simulink model "Tractive_System_model"  (R2025b)
settings: Solver=ode15s  StartTime=0  StopTime=85  MaxStep=1e-5  MinStep=1e-8  RelTol=1e-3  AbsTol=1e-6
undefined symbols (not defined in the file): FL, FR, RL, RR
libraries: batteryecm_lib x280, fl_lib x60, nesl_utility x36, ee_lib x9, sdl_lib x9, simulink x1, slpidlib x1, autolibshared x1, eePmsmFieldOrientedControl x1, eePmsmFwController x1
(part 23 of 23)

== system Tractive_System_model/Electric Powertrain/Scopes Motor/losses ==
  idq : Inport
  w : Inport  Port=2
  Constant : Constant  Value=666.7
  Constant1 : Constant  Value=0.0393
  Constant2 : Constant  Value=[0.695, 8.35e-4, 5.37e-3]  OutDataTypeStr=double
  Constant3 : Constant  Value=[0.298, 3.58e-4, 2.30e-3]  OutDataTypeStr=double
  MATLAB Function : MATLAB Function  TreatAsAtomicUnit=on
  tq_loss : Outport
  wires:
  w/1 -> MATLAB Function/2(w)
  MATLAB Function/1(trq_loss) -> tq_loss/1
  idq/1 -> MATLAB Function/1(idq)
  Constant/1 -> MATLAB Function/4(f_losses)
  Constant1/1 -> MATLAB Function/3(PM)
  Constant2/1 -> MATLAB Function/5(losses_oc)
  Constant3/1 -> MATLAB Function/6(losses_sc)

== system Tractive_System_model/Electric Powertrain/Thermal model/Sensing Temperature Rot ==
  PS-Simulink Converter : nesl_utility/PS-Simulink Converter  PhysicalDomain=network_engine_domain  SubClassName=ps_output  LeftPortType=input  RightPortType=output  PseudoPeriodic=off  Frequencies=[]  VectorFormat=1-D array  Unit=degC  AffineConversion=on
  Temperature Sensor : fl_lib/Thermal/Thermal Sensors/Temperature Sensor  temperature_measure=foundation.enum.MeasurementReference.difference
  ThRef : fl_lib/Thermal/Thermal Elements/Thermal Reference
  H : PMIOPort  Side=Left
  tag scope: TR=global
  wires:
  PS-Simulink Converter/1 -> [TR]
  connections:
  Temperature Sensor/RConn2 -- PS-Simulink Converter/LConn1
  ThRef/LConn1 -- Temperature Sensor/RConn1
  H/RConn1 -- Temperature Sensor/LConn1

== system Tractive_System_model/Electric Powertrain/Thermal model/Sensing Temperature WiA ==
  PS-Simulink Converter : nesl_utility/PS-Simulink Converter  PhysicalDomain=network_engine_domain  SubClassName=ps_output  LeftPortType=input  RightPortType=output  PseudoPeriodic=off  Frequencies=[]  VectorFormat=1-D array  Unit=degC  AffineConversion=on
  Temperature Sensor : fl_lib/Thermal/Thermal Sensors/Temperature Sensor  temperature_measure=foundation.enum.MeasurementReference.difference
  ThRef : fl_lib/Thermal/Thermal Elements/Thermal Reference
  H : PMIOPort  Side=Left
  tag scope: TA=global
  wires:
  PS-Simulink Converter/1 -> [TA]
  connections:
  H/RConn1 -- Temperature Sensor/LConn1
  ThRef/LConn1 -- Temperature Sensor/RConn1
  Temperature Sensor/RConn2 -- PS-Simulink Converter/LConn1

== system Tractive_System_model/Electric Powertrain/Thermal model/Sensing Temperature WiB ==
  PS-Simulink Converter : nesl_utility/PS-Simulink Converter  PhysicalDomain=network_engine_domain  SubClassName=ps_output  LeftPortType=input  RightPortType=output  PseudoPeriodic=off  Frequencies=[]  VectorFormat=1-D array  Unit=degC  AffineConversion=on
  Temperature Sensor : fl_lib/Thermal/Thermal Sensors/Temperature Sensor  temperature_measure=foundation.enum.MeasurementReference.difference
  ThRef : fl_lib/Thermal/Thermal Elements/Thermal Reference
  H : PMIOPort  Side=Left
  tag scope: TB=global
  wires:
  PS-Simulink Converter/1 -> [TB]
  connections:
  Temperature Sensor/RConn2 -- PS-Simulink Converter/LConn1
  ThRef/LConn1 -- Temperature Sensor/RConn1
  H/RConn1 -- Temperature Sensor/LConn1

== system Tractive_System_model/Electric Powertrain/Thermal model/Sensing Temperature WiC ==
  PS-Simulink Converter : nesl_utility/PS-Simulink Converter  PhysicalDomain=network_engine_domain  SubClassName=ps_output  LeftPortType=input  RightPortType=output  PseudoPeriodic=off  Frequencies=[]  VectorFormat=1-D array  Unit=degC  AffineConversion=on
  Temperature Sensor : fl_lib/Thermal/Thermal Sensors/Temperature Sensor  temperature_measure=foundation.enum.MeasurementReference.difference
  ThRef : fl_lib/Thermal/Thermal Elements/Thermal Reference
  H : PMIOPort  Side=Left
  tag scope: TC=global
  wires:
  PS-Simulink Converter/1 -> [TC]
  connections:
  H/RConn1 -- Temperature Sensor/LConn1
  ThRef/LConn1 -- Temperature Sensor/RConn1
  Temperature Sensor/RConn2 -- PS-Simulink Converter/LConn1

== system Tractive_System_model/Electric Powertrain/Vbus/Subsystem2 ==
  Bus Voltage : nesl_utility/PS-Simulink Converter  PhysicalDomain=network_engine_domain  SubClassName=ps_output  LeftPortType=input  RightPortType=output  PseudoPeriodic=off  Frequencies=[]  VectorFormat=inherit  Unit=inherit  AffineConversion=off
  Scope : Scope
      settings: ActiveDisplayYMinimum=569.55394508552229  ActiveDisplayYMaximum=572.89837899883594  DataLoggingVariableName=ScopeData2
  Voltage Sensor : fl_lib/Electrical/Electrical Sensors/Voltage Sensor
  Conn1 : PMIOPort  Side=Right
  Conn2 : PMIOPort  Port=2  Side=Left
  Out1 : Outport
  wires:
  Bus Voltage/1 -> Out1/1, Scope/1
  connections:
  Voltage Sensor/RConn2 -- Conn1/RConn1
  Voltage Sensor/LConn1 -- Conn2/RConn1
  Bus Voltage/LConn1 -- Voltage Sensor/RConn1

== system Tractive_System_model/Longitudinal Vehicle Dynamics/Brakes/Sensing FL ==
  Mechanical Rotational Reference : fl_lib/Mechanical/Rotational Elements/Mechanical Rotational Reference
  Motion Sensor : fl_lib/Mechanical/Mechanical Sensors/Ideal Rotational Motion Sensor  reference=foundation.enum.MeasurementReference.difference  acceleration_port=false  velocity_port=true  position_port=true  wrap_angle=simscape.enum.onoff.off  offset=0 rad
  PS Terminator : fl_lib/Physical Signals/Sinks/PS Terminator
  PS-Simulink Converter : nesl_utility/PS-Simulink Converter  PhysicalDomain=network_engine_domain  SubClassName=ps_output  LeftPortType=input  RightPortType=output  PseudoPeriodic=off  Frequencies=[]  VectorFormat=inherit  Unit=inherit  AffineConversion=off
  PS-Simulink Converter1 : nesl_utility/PS-Simulink Converter  PhysicalDomain=network_engine_domain  SubClassName=ps_output  LeftPortType=input  RightPortType=output  PseudoPeriodic=off  Frequencies=[]  VectorFormat=inherit  Unit=inherit  AffineConversion=off
  Torque Sensor : fl_lib/Mechanical/Mechanical Sensors/Ideal Torque Sensor
  C : PMIOPort  Side=Left
  R : PMIOPort  Port=2  Side=Right
  Out Bus Element : Outport  PortName=m  Element=brkTrqFL
  Out Bus Element1 : Outport  PortName=m  Element=wFL
  wires:
  PS-Simulink Converter1/1 -> Out Bus Element1/1  "w"
  PS-Simulink Converter/1 -> Out Bus Element/1  "trq"
  connections:
  Motion Sensor/RConn3 -- PS Terminator/LConn1
  PS-Simulink Converter1/LConn1 -- Motion Sensor/RConn2
  Motion Sensor/RConn1 -- Mechanical Rotational Reference/LConn1
  Torque Sensor/RConn1 -- C/RConn1
  Motion Sensor/LConn1 -- Torque Sensor/LConn1 -- R/RConn1
  PS-Simulink Converter/LConn1 -- Torque Sensor/RConn2

== system Tractive_System_model/Longitudinal Vehicle Dynamics/Brakes/Sensing FR ==
  Mechanical Rotational Reference : fl_lib/Mechanical/Rotational Elements/Mechanical Rotational Reference
  Motion Sensor : fl_lib/Mechanical/Mechanical Sensors/Ideal Rotational Motion Sensor  reference=foundation.enum.MeasurementReference.difference  acceleration_port=false  velocity_port=true  position_port=true  wrap_angle=simscape.enum.onoff.off  offset=0 rad
  PS Terminator : fl_lib/Physical Signals/Sinks/PS Terminator
  PS-Simulink Converter : nesl_utility/PS-Simulink Converter  PhysicalDomain=network_engine_domain  SubClassName=ps_output  LeftPortType=input  RightPortType=output  PseudoPeriodic=off  Frequencies=[]  VectorFormat=inherit  Unit=inherit  AffineConversion=off
  PS-Simulink Converter1 : nesl_utility/PS-Simulink Converter  PhysicalDomain=network_engine_domain  SubClassName=ps_output  LeftPortType=input  RightPortType=output  PseudoPeriodic=off  Frequencies=[]  VectorFormat=inherit  Unit=inherit  AffineConversion=off
  Torque Sensor : fl_lib/Mechanical/Mechanical Sensors/Ideal Torque Sensor
  C : PMIOPort  Side=Left
  R : PMIOPort  Port=2  Side=Right
  Out Bus Element : Outport  PortName=m  Element=brkTrqFR
  Out Bus Element1 : Outport  PortName=m  Element=wFR
  wires:
  PS-Simulink Converter/1 -> Out Bus Element/1  "trq"
  PS-Simulink Converter1/1 -> Out Bus Element1/1  "w"
  connections:
  PS-Simulink Converter/LConn1 -- Torque Sensor/RConn2
  R/RConn1 -- Torque Sensor/LConn1 -- Motion Sensor/LConn1
  Torque Sensor/RConn1 -- C/RConn1
  Motion Sensor/RConn1 -- Mechanical Rotational Reference/LConn1
  PS-Simulink Converter1/LConn1 -- Motion Sensor/RConn2
  Motion Sensor/RConn3 -- PS Terminator/LConn1

== system Tractive_System_model/Longitudinal Vehicle Dynamics/Brakes/Sensing RL ==
  Mechanical Rotational Reference : fl_lib/Mechanical/Rotational Elements/Mechanical Rotational Reference
  Motion Sensor : fl_lib/Mechanical/Mechanical Sensors/Ideal Rotational Motion Sensor  reference=foundation.enum.MeasurementReference.difference  acceleration_port=false  velocity_port=true  position_port=true  wrap_angle=simscape.enum.onoff.off  offset=0 rad
  PS Terminator : fl_lib/Physical Signals/Sinks/PS Terminator
  PS-Simulink Converter : nesl_utility/PS-Simulink Converter  PhysicalDomain=network_engine_domain  SubClassName=ps_output  LeftPortType=input  RightPortType=output  PseudoPeriodic=off  Frequencies=[]  VectorFormat=inherit  Unit=inherit  AffineConversion=off
  PS-Simulink Converter1 : nesl_utility/PS-Simulink Converter  PhysicalDomain=network_engine_domain  SubClassName=ps_output  LeftPortType=input  RightPortType=output  PseudoPeriodic=off  Frequencies=[]  VectorFormat=inherit  Unit=inherit  AffineConversion=off
  Torque Sensor : fl_lib/Mechanical/Mechanical Sensors/Ideal Torque Sensor
  C : PMIOPort  Side=Left
  R : PMIOPort  Port=2  Side=Right
  Out Bus Element : Outport  PortName=m  Element=brkTrqRL
  Out Bus Element1 : Outport  PortName=m  Element=wRL
  wires:
  PS-Simulink Converter/1 -> Out Bus Element/1  "trq"
  PS-Simulink Converter1/1 -> Out Bus Element1/1  "w"
  connections:
  PS-Simulink Converter/LConn1 -- Torque Sensor/RConn2
  Torque Sensor/LConn1 -- Motion Sensor/LConn1 -- R/RConn1
  Torque Sensor/RConn1 -- C/RConn1
  Motion Sensor/RConn1 -- Mechanical Rotational Reference/LConn1
  PS-Simulink Converter1/LConn1 -- Motion Sensor/RConn2
  Motion Sensor/RConn3 -- PS Terminator/LConn1

== system Tractive_System_model/Longitudinal Vehicle Dynamics/Chassis and Tires/Subsystem ==
  PS-Simulink Converter : nesl_utility/PS-Simulink Converter  PhysicalDomain=network_engine_domain  SubClassName=ps_output  LeftPortType=input  RightPortType=output  PseudoPeriodic=off  Frequencies=[]  VectorFormat=inherit  Unit=inherit  AffineConversion=off
  Torque Sensor Motor RL : fl_lib/Mechanical/Mechanical Sensors/Ideal Torque Sensor
  C : PMIOPort  Side=Left
  R : PMIOPort  Port=2  Side=Right
  T : Outport
  wires:
  PS-Simulink Converter/1 -> T/1
  connections:
  Torque Sensor Motor RL/RConn1 -- C/RConn1
  Torque Sensor Motor RL/LConn1 -- R/RConn1
  PS-Simulink Converter/LConn1 -- Torque Sensor Motor RL/RConn2

== system Tractive_System_model/Longitudinal Vehicle Dynamics/Chassis and Tires/Subsystem1 ==
  PS-Simulink Converter : nesl_utility/PS-Simulink Converter  PhysicalDomain=network_engine_domain  SubClassName=ps_output  LeftPortType=input  RightPortType=output  PseudoPeriodic=off  Frequencies=[]  VectorFormat=inherit  Unit=inherit  AffineConversion=off
  Torque Sensor Motor RL : fl_lib/Mechanical/Mechanical Sensors/Ideal Torque Sensor
  C : PMIOPort  Side=Left
  R : PMIOPort  Port=2  Side=Right
  T : Outport
  wires:
  PS-Simulink Converter/1 -> T/1
  connections:
  PS-Simulink Converter/LConn1 -- Torque Sensor Motor RL/RConn2
  Torque Sensor Motor RL/LConn1 -- R/RConn1
  Torque Sensor Motor RL/RConn1 -- C/RConn1

== matlab function Tractive_System_model/Electric Powertrain/Scopes Motor/losses/MATLAB Function ==
  data: idq input; w input; PM input; f_losses input; losses_oc input; losses_sc input; trq_loss output
function trq_loss = losses(idq, w, PM, f_losses, losses_oc, losses_sc)
    % =========================================================
    % Iron Loss Torque Loss Model for EMRAX 208 PMSM
    % Inputs:
    %   idq       - [id, iq] dq-axis currents [A] (2x1 vector)
    %   w         - Rotor angular velocity [rad/s]
    %   PM        - Permanent magnet flux linkage [Vs] = 0.0393
    %   f_losses  - Base electrical frequency [Hz] = 666.7
    %   losses_oc - Open circuit loss coefficients [a_h, a_J, a_ex]
    %               = [0.695, 8.35e-4, 5.37e-3]
    %   losses_sc - Short circuit loss coefficients [b_h, b_J, b_ex]
    %               = [0.298, 3.58e-4, 2.30e-3]
    % Output:
    %   trq_loss  - Torque loss due to iron losses [Nm]
    % =========================================================

    % --- Constants & Parameters ---
    N          = 10;    % Number of pole pairs (EMRAX 208)
    Isc_losses = 100;   % Short-circuit RMS current [A]

    % --- Demux idq input ---
    i_d = idq(1);
    i_q = idq(2);

    % --- Step 1: Flux Linkage ---
    lambda = PM;        % Already in Vs/Wb, no conversion needed

    % --- Step 2: Open-Circuit Loss Coefficients (Main Flux) ---
    a_h  = losses_oc(1) / f_losses;
    a_J  = losses_oc(2) / f_losses^2;
    a_ex = losses_oc(3) / f_losses^1.5;

    % --- Step 3: Short-Circuit Loss Coefficients (Cross-Tooth Flux) ---
    b_h  = losses_sc(1) / f_losses;
    b_J  = losses_sc(2) / f_losses^2;
    b_ex = losses_sc(3) / f_losses^1.5;

    % --- Step 4: Current Normalisation ---
    Id    = abs(i_d) / sqrt(2);
    Iq    = abs(i_q) / sqrt(2);
    w_abs = abs(w);

    % --- Step 5: Cap Id ratio to prevent singularity ---
    ratio_Id_Isc = min(Id / Isc_losses, 0.999);

    % --- Step 6: Voltage Proxies for Iron Losses ---
    Vd = lambda * w_abs * N / (2*pi) * ratio_Id_Isc;

    Vm = lambda * w_abs * N / (2*pi) * ...
         sqrt((1 - ratio_Id_Isc)^2 + (Iq / Isc_losses)^2);

    % --- Step 7: Power Loss Calculation ---
    Vm_losses = (a_h  / lambda      ) * Vm   + ...
                (a_J  / lambda^2    ) * Vm^2 + ...
                (a_ex / lambda^1.5  ) * Vm^1.5;

    Vd_losses = (b_h  / lambda      ) * Vd   + ...
                (b_J  / lambda^2    ) * Vd^2 + ...
                (b_ex / lambda^1.5  ) * Vd^1.5;

    % --- Step 8: Torque Loss Conversion ---
    % Protected against division by zero at w = 0
    if w_abs < 0.01
        trq_loss = 0;
    else
        trq_loss = sign(w) * (Vd_losses + Vm_losses) / w_abs;
    end

end
